simulink model "desarrollo"  (R2021a)
settings: Solver=VariableStepAuto  StartTime=0.0  StopTime=4  RelTol=1e-3
values from neighbouring files (symbols this model uses):
  den = conv([L R],[J b]);den(1,end)=den(1,end)+K*K    [desarrollo.m]    (also in pr1.m = conv(den,1/0.3))
  num = K    (= 0.01)    [desarrollo.m]    (also in pr1.m = 166.666666667)
settings Model: Creator=pierr  LastModifiedBy=pierr

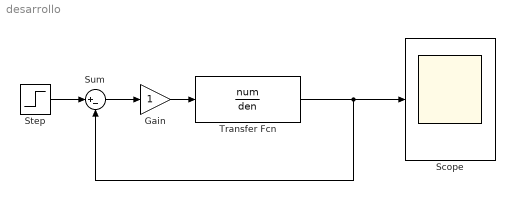
== system desarrollo ==
  Gain : Gain
  Scope : Scope
  Step : Step  Time=0  After=10  SampleTime=0
  Sum : Sum  Inputs=|+-
  Transfer Fcn : TransferFcn  Numerator=num  Denominator=den
  wires:
  Transfer Fcn/1 -> Sum/2, Scope/1
  Gain/1 -> Transfer Fcn/1
  Sum/1 -> Gain/1
  Step/1 -> Sum/1
